simulink model "HealthResultEncoder"  (R2023a)
settings: Solver=VariableStepAuto  StartTime=0.0  StopTime=10.0  RelTol=1e-3
undefined symbols (not defined in the file): I, OIn
settings Model: Creator=aan18022  LastModifiedBy=aan18022

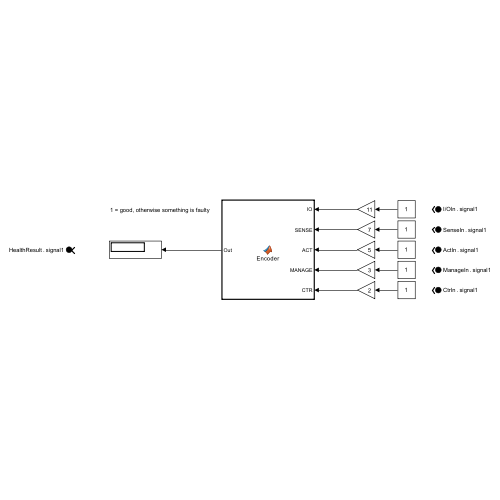
[thumbnail: Simulink's stored preview of the top-level diagram]
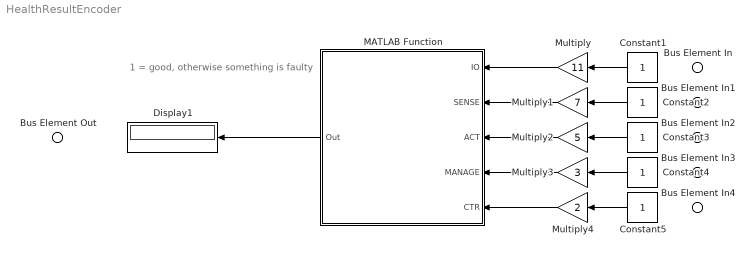
== system HealthResultEncoder ==
  note: 1 = good, otherwise something is faulty
  Bus Element In : Inport  PortName=I/OIn  Element=signal1
  Bus Element In1 : Inport  Port=2  PortName=SenseIn  Element=signal1
  Bus Element In2 : Inport  Port=3  PortName=ActIn  Element=signal1
  Bus Element In3 : Inport  Port=4  PortName=ManageIn  Element=signal1
  Bus Element In4 : Inport  Port=5  PortName=CtrIn  Element=signal1
  Constant{1..5} (5 alike) : Constant
  Display1 : Display
  MATLAB Function : MATLAB Function  TreatAsAtomicUnit=on
  Multiply : Gain  Gain=11
  Multiply1 : Gain  Gain=7
  Multiply2 : Gain  Gain=5
  Multiply3 : Gain  Gain=3
  Multiply4 : Gain  Gain=2
  Bus Element Out : Outport  PortName=HealthResult  Element=signal1
  wires:
  Multiply/1 -> MATLAB Function/1(IO)
  Multiply1/1 -> MATLAB Function/2(SENSE)
  Multiply2/1 -> MATLAB Function/3(ACT)
  Multiply3/1 -> MATLAB Function/4(MANAGE)
  Multiply4/1 -> MATLAB Function/5(CTR)
  Constant1/1 -> Multiply/1
  Constant2/1 -> Multiply1/1
  Constant3/1 -> Multiply2/1
  Constant4/1 -> Multiply3/1
  Constant5/1 -> Multiply4/1
  MATLAB Function/1(Out) -> Display1/1

== matlab function HealthResultEncoder/MATLAB Function ==
  data: IO input; Out output; SENSE input; ACT input; MANAGE input; CTR input
function Out= Encoder(IO,SENSE,ACT,MANAGE,CTR)

if IO == 0
    io = 1;
else
    io = IO;
end

if SENSE == 0
    sense = 1;
else
    sense = SENSE;
end

if ACT == 0
    act = 1;
else
    act = ACT;
end

if MANAGE == 0
    manage = 1;
else
    manage = MANAGE;
end

if CTR == 0
    ctr = 1;
else
    ctr = CTR;
end

Out = io * sense * act * manage * ctr;
